simulink library "tetherInternalForcesNGreater2_ul"  (R2018b)
settings: Solver=VariableStepAuto  StartTime=0.0  StopTime=10.0  RelTol=1e-3
values from neighbouring files (symbols this model uses):
  dia_t = 0.01    [tetherInternalForces_ts.m]
  E = 3.8e9    (= 3800000000)    [tetherInternalForces_ts.m]
  mass = 100    [tetherInternalForces_ts.m]
  N = 4    [tetherInternalForces_ts.m]
  zeta = 0.05    [tetherInternalForces_ts.m]
settings Model: Creator=asiddiq2  LastModifiedBy=mcobb

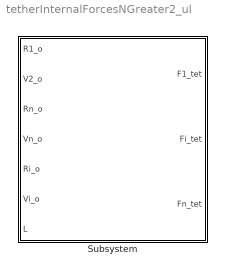
== system tetherInternalForcesNGreater2_ul ==
  Subsystem : Subsystem  mask{N=N, E=E, dia_t=dia_t, mass=mass, zeta=zeta}
      mask prompts: N "Number of nodes (N>=2)"; E "Youngs Modulus (N/m^2)"; dia_t "Tether diameter (m)"; mass "Vehicle Mass (kg)"; zeta "Damping ratio"

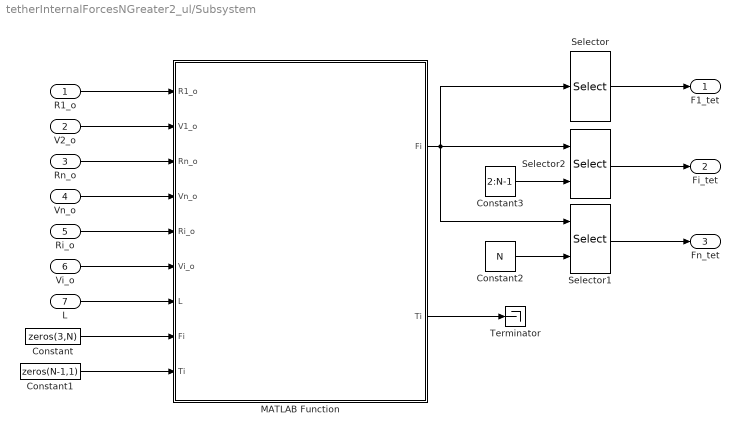
== system tetherInternalForcesNGreater2_ul/Subsystem ==
  R1_o : Inport
  V2_o : Inport  Port=2
  Rn_o : Inport  Port=3
  Vn_o : Inport  Port=4
  Ri_o : Inport  Port=5
  Vi_o : Inport  Port=6
  L : Inport  Port=7
  Constant : Constant  Value=zeros(3,N)
  Constant1 : Constant  Value=zeros(N-1,1)
  Constant2 : Constant  Value=N
  Constant3 : Constant  Value=2:N-1
  MATLAB Function : MATLAB Function  TreatAsAtomicUnit=on
  Selector : Selector  NumberOfDimensions=2  InputPortWidth=3  IndexOptions=Select all,Index vector (dialog)  Indices=[1 3],1  OutputSizes=1,1
  Selector1 : Selector  NumberOfDimensions=2  InputPortWidth=3  IndexOptions=Select all,Index vector (port)  Indices=[1 3],N  OutputSizes=1,1
  Selector2 : Selector  NumberOfDimensions=2  InputPortWidth=3  IndexOptions=Select all,Index vector (port)  Indices=[1 3],[2:N-1]  OutputSizes=1,1
  Terminator : Terminator
  F1_tet : Outport
  Fi_tet : Outport  Port=2
  Fn_tet : Outport  Port=3
  wires:
  MATLAB Function/2(Ti) -> Terminator/1
  Rn_o/1 -> MATLAB Function/3(Rn_o)
  Vn_o/1 -> MATLAB Function/4(Vn_o)
  Ri_o/1 -> MATLAB Function/5(Ri_o)
  Vi_o/1 -> MATLAB Function/6(Vi_o)
  R1_o/1 -> MATLAB Function/1(R1_o)
  V2_o/1 -> MATLAB Function/2(V1_o)
  L/1 -> MATLAB Function/7(L)
  Constant/1 -> MATLAB Function/8("Fi ")
  Constant1/1 -> MATLAB Function/9("Ti ")
  Selector/1 -> F1_tet/1
  Selector1/1 -> Fn_tet/1
  Selector2/1 -> Fi_tet/1
  MATLAB Function/1(Fi) -> Selector2/1, Selector1/1, Selector/1
  Constant2/1 -> Selector1/2
  Constant3/1 -> Selector2/2

== matlab function tetherInternalForcesNGreater2_ul/Subsystem/MATLAB Function ==
  data: R1_o input; V1_o input; Rn_o input; Vn_o input; Fi output; Ri_o input; Vi_o input; L input; Fi input; Ti input; N parameter; mass parameter; zeta parameter; dia_t parameter; E parameter; Ti output
 function [Fi,Ti]  = fcn(R1_o,V1_o,Rn_o,Vn_o,Ri_o,Vi_o,L,Fi,Ti,N, mass, zeta, dia_t, E)

Ri_o = [R1_o Ri_o Rn_o];
Vi_o = [V1_o Vi_o Vn_o];
 
% cross sectional area
CS = (pi/4)*dia_t^2;

% total spring stiffness
k_tot = E*CS/L;

% total damping coefficient
c_tot = zeta*2*sqrt(k_tot*mass);

% inidividual spring stiffness and damping
k = k_tot*(N-1);
c = c_tot*(N-1);
Li = L/(N-1);

% determine distance between nodes and the derivatives of each element
di = zeros(N-1,1);
direction = zeros(3,N-1);
di_dot = zeros(N-1,1);
Tk = zeros(N-1,1);
Td = zeros(N-1,1);
F_t_i = zeros(3,N);


for ii = 1:N-1
        di(ii) = norm(Ri_o(:,ii+1) - Ri_o(:,ii));
        direction(:,ii) = (Ri_o(:,ii+1) - Ri_o(:,ii))/di(ii);
        di_dot(ii) = dot(Ri_o(:,ii+1) - Ri_o(:,ii),Vi_o(:,ii+1) - Vi_o(:,ii))/di(ii);
    
end

% spring and damper forces
for ii = 1:N-1
    if di(ii) > Li
        Tk(ii) = k*(di(ii) - Li);
        Td(ii) = c*di_dot(ii);
        F_t_i(:,ii) = (Tk(ii) + Td(ii))*direction(:,ii);
        Ti(ii) = norm(F_t_i(:,ii));
    else
        Tk(ii) = 0;
        Td(ii) = 0;
        F_t_i(:,ii) = (Tk(ii) + Td(ii))*direction(:,ii);
        Ti(ii) = norm(F_t_i(:,ii));

    end
end

for ii = 1:N
    if ii == 1
        Fi(:,ii) = F_t_i(:,ii);
    elseif ii > 1 && ii < N
        Fi(:,ii) = F_t_i(:,ii) - F_t_i(:,ii-1);
    elseif ii == N
        Fi(:,ii) = -F_t_i(:,ii-1);
    end
end


% Mitchells version here (Should be equivalen to almost all of the above)
%  di = sqrt(sum(diff(Ri_o,1,2).^2,1))';
%  direction = diff(Ri_o,1,2)./repmat(di',[N-1 1]);
%  di_dot = sum(direction.*diff(Vi_o,1,2),1)';
%  Tk(di>Li) = k*(di(di>Li) - Li)
%  Td(di>Li) = c*di_dot(di>Li)
%  F_t_i(1:end-1) = repmat((Tk' + Td'),[N-1 1]).*direction


end
